simulink model "ultra"  (R2020b)
settings: Solver=FixedStepDiscrete  StartTime=0.0  StopTime=10.0  FixedStep=0.0005  RelTol=1e-3  EnableMultiTasking=on
undefined symbols (not defined in the file): acc_calmax1, acc_calmax2, acc_calmin1, acc_calmin2, akemancanshu, bre, bre_calmax, bre_calmin, ecucoder_acal, I_AN01_5K1, I_AN03_5V, I_AN04_5V, kd, ki, kp, leftmax, O_SW06_HS1A, rightmax, T_add, T_del, tiaoshi, zhiling
libraries: ec5744lib x215, canmsglib x75, simulink x10
(part 3 of 7)

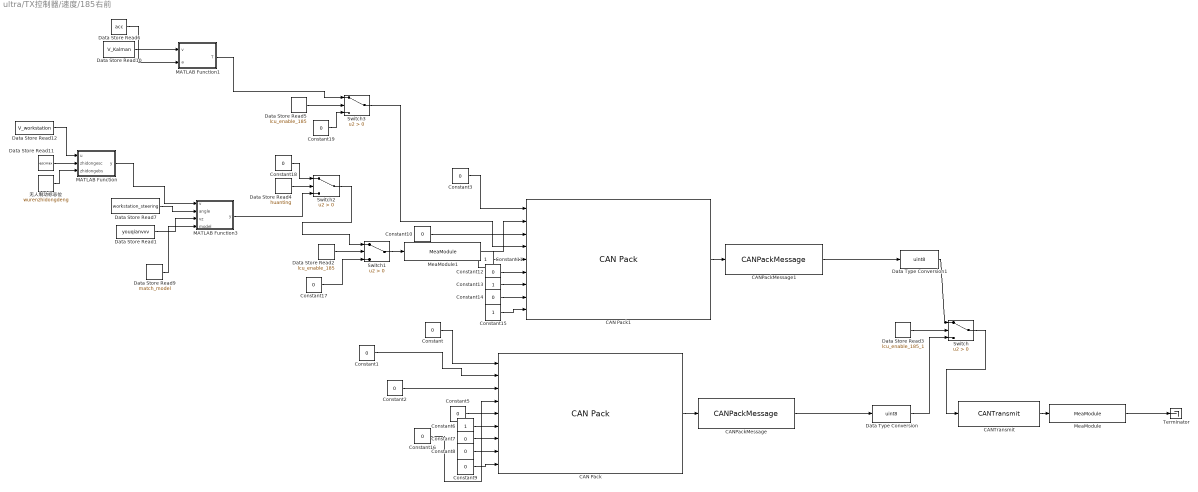
== system ultra/TX控制器/速度/185右前 ==
  CAN Pack : canmsglib/CAN Pack  CANdbFile=D:\desktop\CANdbc\enable - youqian.dbc  MsgList=(none)  MsgName=first_enable  MsgIDType=Standard (11-bit identifier)  MsgIdentifier=389  MsgLength=8  Remote=off  ApplyMinMax=off  BusOutput=off  SignalInfo={'AMK_Reserve','12','4','LE','signed','Standard','0','1','0','0','15';'AMK_TargetVelocity','16','16','LE','signed','Standard','0','1','0','0','65535';'AMK_TorqueLimitNegativ','48','16','LE','signed','Standard','0','1','0','0','65535';'AMK_TorqueLimitPositiv','32','16','LE','signed','Standard','0','1','0','0','65535';'AMK_bEnable','10','1','LE','unsigned','Standard','0','1','0','0','1';'AMK_bErrorReset','11','1','LE','unsigned','Standard','0','1','0','0','1';'AMK_bInverterOn','8','1','LE','unsigned','Standard','0','1','0','0','1';'AMK_bReserve','0','8','LE','unsigned','Standard','0','1','0','0','255';'CAN_bdcon','9','1','LE','unsigned','Standard','0','1','0','0','1'}
      settings: SourceProductBaseCode=ME,XP,VN  DataFormat=CANdb specified signals
  CAN Pack1 : canmsglib/CAN Pack  CANdbFile=D:\desktop\CANdbc\enable - youqian.dbc  MsgList=(none)  MsgName=first_enable  MsgIDType=Standard (11-bit identifier)  MsgIdentifier=389  MsgLength=8  Remote=off  ApplyMinMax=off  BusOutput=off  SignalInfo={'AMK_Reserve','12','4','LE','signed','Standard','0','1','0','0','15';'AMK_TargetVelocity','16','16','LE','signed','Standard','0','1','0','0','65535';'AMK_TorqueLimitNegativ','48','16','LE','signed','Standard','0','1','0','0','65535';'AMK_TorqueLimitPositiv','32','16','LE','signed','Standard','0','1','0','0','65535';'AMK_bEnable','10','1','LE','unsigned','Standard','0','1','0','0','1';'AMK_bErrorReset','11','1','LE','unsigned','Standard','0','1','0','0','1';'AMK_bInverterOn','8','1','LE','unsigned','Standard','0','1','0','0','1';'AMK_bReserve','0','8','LE','unsigned','Standard','0','1','0','0','255';'CAN_bdcon','9','1','LE','unsigned','Standard','0','1','0','0','1'}
      settings: SourceProductBaseCode=ME,XP,VN  DataFormat=CANdb specified signals
  CANPackMessage : ec5744lib/RapidECU_U4B/04CANCommunication/CANPackMessage  datalength=8  sampletime=-1
      settings: SourceProductName=ECUCoder for MPC5744
  CANPackMessage1 : ec5744lib/RapidECU_U4B/04CANCommunication/CANPackMessage  datalength=8  sampletime=-1
      settings: SourceProductName=ECUCoder for MPC5744
  CANTransmit : ec5744lib/RapidECU_U4B/04CANCommunication/CANTransmit  canmodule=0  canbuffer=11  canmessageid=hex2dec('185')  canmessagetype=Standard(11-bit ID)  datalength=8  sampletime=-1
      settings: SourceProductName=ECUCoder for MPC5744
  Constant{,1..3,5,7..10,12,14,16..17,19} (14 alike) : Constant  Value=0  SampleTime=-1
  Constant{6,11,13,15} (4 alike) : Constant  SampleTime=-1
  Constant18 : Constant  Value=0
  Data Store Read1 : DataStoreRead  DataStoreName=youqianvvv
  Data Store Read10 : DataStoreRead  DataStoreName=V_Kalman
  Data Store Read11 : DataStoreRead  DataStoreName=escmax
  Data Store Read12 : DataStoreRead  DataStoreName=V_workstation
  Data Store Read2 : DataStoreRead  DataStoreName=lcu_enable_185
  Data Store Read3 : DataStoreRead  DataStoreName=lcu_enable_185_1
  Data Store Read4 : DataStoreRead  DataStoreName=huanting
  Data Store Read5 : DataStoreRead  DataStoreName=lcu_enable_185
  Data Store Read6 : DataStoreRead  DataStoreName=acc
  Data Store Read7 : DataStoreRead  DataStoreName=workstation_steering
  Data Store Read9 : DataStoreRead  DataStoreName=match_model
  Data Type Conversion : DataTypeConversion  OutDataTypeStr=uint8
  Data Type Conversion1 : DataTypeConversion  OutDataTypeStr=uint8
  MATLAB Function : MATLAB Function  TreatAsAtomicUnit=on
  MATLAB Function1 : MATLAB Function  TreatAsAtomicUnit=on
  MATLAB Function3 : MATLAB Function  TreatAsAtomicUnit=on
  MeaModule : ec5744lib/RapidECU_U4B/07Calibration/MeaModule  signal=V185
      settings: SourceProductName=ECUCoder for MPC5744
  MeaModule1 : ec5744lib/RapidECU_U4B/07Calibration/MeaModule  signal=Vforth
      settings: SourceProductName=ECUCoder for MPC5744
  Switch{,1..3} (4 alike) : Switch  Criteria=u2 > Threshold
  Terminator : Terminator
  无人制动标志位 : DataStoreRead  DataStoreName=wurenzhidongdeng
  wires:
  Constant8/1 -> CAN Pack/8
  Constant5/1 -> CAN Pack/5
  Constant/1 -> CAN Pack/1
  CANPackMessage/1 -> Data Type Conversion/1
  Constant9/1 -> CAN Pack/9
  CAN Pack/1 -> CANPackMessage/1
  Constant7/1 -> CAN Pack/7
  Constant1/1 -> CAN Pack/2
  Constant16/1 -> CAN Pack/4
  Constant2/1 -> CAN Pack/3
  Constant6/1 -> CAN Pack/6
  CANTransmit/1 -> MeaModule/1
  MeaModule/1 -> Terminator/1
  CANPackMessage1/1 -> Data Type Conversion1/1
  Constant3/1 -> CAN Pack1/1
  Constant11/1 -> CAN Pack1/5
  Constant12/1 -> CAN Pack1/6
  Constant13/1 -> CAN Pack1/7
  CAN Pack1/1 -> CANPackMessage1/1
  Constant10/1 -> CAN Pack1/3
  Constant14/1 -> CAN Pack1/8
  Constant15/1 -> CAN Pack1/9
  Data Type Conversion1/1 -> Switch/1
  Data Type Conversion/1 -> Switch/3
  Switch/1 -> CANTransmit/1
  Data Store Read3/1 -> Switch/2
  Switch1/1 -> MeaModule1/1
  Constant17/1 -> Switch1/3
  Data Store Read2/1 -> Switch1/2
  Data Store Read4/1 -> Switch2/2
  Constant18/1 -> Switch2/1
  Switch2/1 -> Switch1/1
  MeaModule1/1 -> CAN Pack1/2
  Constant19/1 -> Switch3/3
  Switch3/1 -> CAN Pack1/4
  Data Store Read5/1 -> Switch3/2
  Data Store Read7/1 -> MATLAB Function3/2(angle)
  Data Store Read1/1 -> MATLAB Function3/3(vz)
  MATLAB Function3/1(y) -> Switch2/3
  Data Store Read9/1 -> MATLAB Function3/4(model)
  MATLAB Function1/1(T) -> Switch3/1
  Data Store Read6/1 -> MATLAB Function1/2(a)
  Data Store Read10/1 -> MATLAB Function1/1(v)
  无人制动标志位/1 -> MATLAB Function/3(zhidongebs)
  MATLAB Function/1(y) -> MATLAB Function3/1(v)
  Data Store Read11/1 -> MATLAB Function/2(zhidongesc)
  Data Store Read12/1 -> MATLAB Function/1(u)

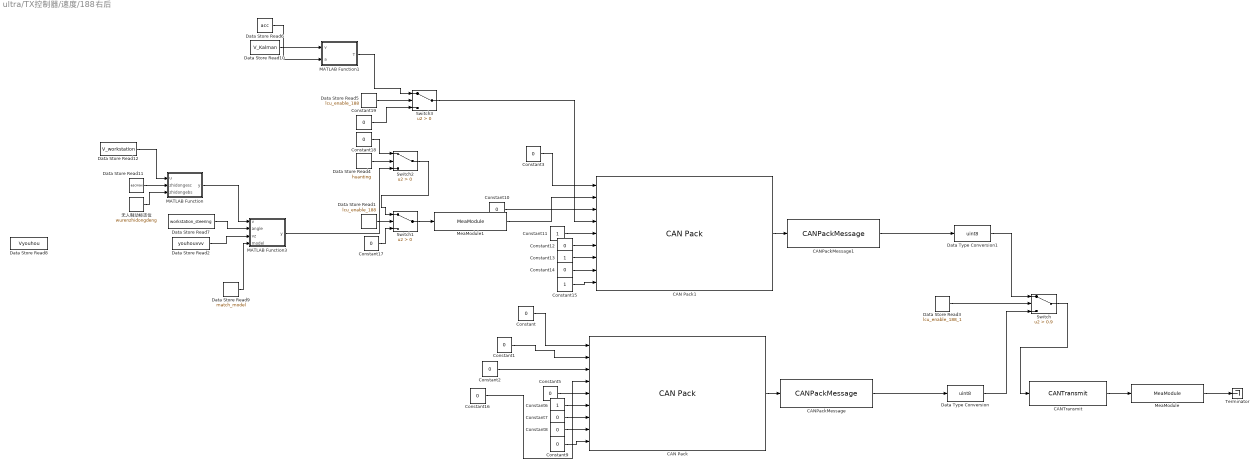
== system ultra/TX控制器/速度/188右后 ==
  CAN Pack : canmsglib/CAN Pack  CANdbFile=D:\desktop\CANdbc\enable - zuohou - 副本.dbc  MsgList=(none)  MsgName=first_enable  MsgIDType=Standard (11-bit identifier)  MsgIdentifier=392  MsgLength=8  Remote=off  ApplyMinMax=off  BusOutput=off  SignalInfo={'AMK_Reserve','12','4','LE','signed','Standard','0','1','0','0','15';'AMK_TargetVelocity','16','16','LE','signed','Standard','0','1','0','0','65535';'AMK_TorqueLimitNegativ','48','16','LE','signed','Standard','0','1','0','0','65535';'AMK_TorqueLimitPositiv','32','16','LE','signed','Standard','0','1','0','0','65535';'AMK_bEnable','10','1','LE','unsigned','Standard','0','1','0','0','1';'AMK_bErrorReset','11','1','LE','unsigned','Standard','0','1','0','0','1';'AMK_bInverterOn','8','1','LE','unsigned','Standard','0','1','0','0','1';'AMK_bReserve','0','8','LE','unsigned','Standard','0','1','0','0','255';'CAN_bdcon','9','1','LE','unsigned','Standard','0','1','0','0','1'}
      settings: SourceProductBaseCode=ME,XP,VN  DataFormat=CANdb specified signals
  CAN Pack1 : canmsglib/CAN Pack  CANdbFile=D:\desktop\CANdbc\enable - zuohou - 副本.dbc  MsgList=(none)  MsgName=first_enable  MsgIDType=Standard (11-bit identifier)  MsgIdentifier=392  MsgLength=8  Remote=off  ApplyMinMax=off  BusOutput=off  SignalInfo={'AMK_Reserve','12','4','LE','signed','Standard','0','1','0','0','15';'AMK_TargetVelocity','16','16','LE','signed','Standard','0','1','0','0','65535';'AMK_TorqueLimitNegativ','48','16','LE','signed','Standard','0','1','0','0','65535';'AMK_TorqueLimitPositiv','32','16','LE','signed','Standard','0','1','0','0','65535';'AMK_bEnable','10','1','LE','unsigned','Standard','0','1','0','0','1';'AMK_bErrorReset','11','1','LE','unsigned','Standard','0','1','0','0','1';'AMK_bInverterOn','8','1','LE','unsigned','Standard','0','1','0','0','1';'AMK_bReserve','0','8','LE','unsigned','Standard','0','1','0','0','255';'CAN_bdcon','9','1','LE','unsigned','Standard','0','1','0','0','1'}
      settings: SourceProductBaseCode=ME,XP,VN  DataFormat=CANdb specified signals
  CANPackMessage : ec5744lib/RapidECU_U4B/04CANCommunication/CANPackMessage  datalength=8  sampletime=-1
      settings: SourceProductName=ECUCoder for MPC5744
  CANPackMessage1 : ec5744lib/RapidECU_U4B/04CANCommunication/CANPackMessage  datalength=8  sampletime=-1
      settings: SourceProductName=ECUCoder for MPC5744
  CANTransmit : ec5744lib/RapidECU_U4B/04CANCommunication/CANTransmit  canmodule=0  canbuffer=9  canmessageid=hex2dec('188')  canmessagetype=Standard(11-bit ID)  datalength=8  sampletime=-1
      settings: SourceProductName=ECUCoder for MPC5744
  Constant{,1..3,5,7..10,12,14,17,19} (13 alike) : Constant  Value=0  SampleTime=-1
  Constant{6,11,13,15} (4 alike) : Constant  SampleTime=-1
  Constant16 : Constant  Value=0
  Constant18 : Constant  Value=0
  Data Store Read1 : DataStoreRead  DataStoreName=lcu_enable_188
  Data Store Read10 : DataStoreRead  DataStoreName=V_Kalman
  Data Store Read11 : DataStoreRead  DataStoreName=escmax
  Data Store Read12 : DataStoreRead  DataStoreName=V_workstation
  Data Store Read2 : DataStoreRead  DataStoreName=youhouvvv
  Data Store Read3 : DataStoreRead  DataStoreName=lcu_enable_188_1
  Data Store Read4 : DataStoreRead  DataStoreName=huanting
  Data Store Read5 : DataStoreRead  DataStoreName=lcu_enable_188
  Data Store Read6 : DataStoreRead  DataStoreName=acc
  Data Store Read7 : DataStoreRead  DataStoreName=workstation_steering
  Data Store Read8 : DataStoreRead  DataStoreName=Vyouhou
  Data Store Read9 : DataStoreRead  DataStoreName=match_model
  Data Type Conversion : DataTypeConversion  OutDataTypeStr=uint8
  Data Type Conversion1 : DataTypeConversion  OutDataTypeStr=uint8
  MATLAB Function : MATLAB Function  TreatAsAtomicUnit=on
  MATLAB Function1 : MATLAB Function  TreatAsAtomicUnit=on
  MATLAB Function3 : MATLAB Function  TreatAsAtomicUnit=on
  MeaModule : ec5744lib/RapidECU_U4B/07Calibration/MeaModule  signal=V188
      settings: SourceProductName=ECUCoder for MPC5744
  MeaModule1 : ec5744lib/RapidECU_U4B/07Calibration/MeaModule  signal=Vsecond
      settings: SourceProductName=ECUCoder for MPC5744
  Switch : Switch  Criteria=u2 > Threshold  Threshold=0.9
  Switch1 : Switch  Criteria=u2 > Threshold
  Switch2 : Switch  Criteria=u2 > Threshold
  Switch3 : Switch  Criteria=u2 > Threshold
  Terminator : Terminator
  无人制动标志位 : DataStoreRead  DataStoreName=wurenzhidongdeng
  wires:
  Constant8/1 -> CAN Pack/8
  Constant5/1 -> CAN Pack/5
  Constant/1 -> CAN Pack/1
  CANPackMessage/1 -> Data Type Conversion/1
  Constant9/1 -> CAN Pack/9
  CAN Pack/1 -> CANPackMessage/1
  Constant7/1 -> CAN Pack/7
  Constant1/1 -> CAN Pack/2
  Constant16/1 -> CAN Pack/4
  Constant2/1 -> CAN Pack/3
  Constant6/1 -> CAN Pack/6
  CANTransmit/1 -> MeaModule/1
  MeaModule/1 -> Terminator/1
  Data Type Conversion1/1 -> Switch/1
  Constant12/1 -> CAN Pack1/6
  Constant10/1 -> CAN Pack1/3
  CANPackMessage1/1 -> Data Type Conversion1/1
  Constant14/1 -> CAN Pack1/8
  Constant3/1 -> CAN Pack1/1
  Constant11/1 -> CAN Pack1/5
  CAN Pack1/1 -> CANPackMessage1/1
  Constant15/1 -> CAN Pack1/9
  Constant13/1 -> CAN Pack1/7
  Data Store Read3/1 -> Switch/2
  Data Type Conversion/1 -> Switch/3
  Switch/1 -> CANTransmit/1
  Constant17/1 -> Switch1/3
  Data Store Read1/1 -> Switch1/2
  Switch1/1 -> MeaModule1/1
  Data Store Read4/1 -> Switch2/2
  Constant18/1 -> Switch2/1
  Switch2/1 -> Switch1/1
  MeaModule1/1 -> CAN Pack1/2
  Switch3/1 -> CAN Pack1/4
  Constant19/1 -> Switch3/3
  Data Store Read5/1 -> Switch3/2
  Data Store Read7/1 -> MATLAB Function3/2(angle)
  MATLAB Function3/1(y) -> Switch2/3
  Data Store Read9/1 -> MATLAB Function3/4(model)
  Data Store Read10/1 -> MATLAB Function1/1(v)
  Data Store Read6/1 -> MATLAB Function1/2(a)
  MATLAB Function1/1(T) -> Switch3/1
  无人制动标志位/1 -> MATLAB Function/3(zhidongebs)
  MATLAB Function/1(y) -> MATLAB Function3/1(v)
  Data Store Read11/1 -> MATLAB Function/2(zhidongesc)
  Data Store Read12/1 -> MATLAB Function/1(u)
  Data Store Read2/1 -> MATLAB Function3/3(vz)

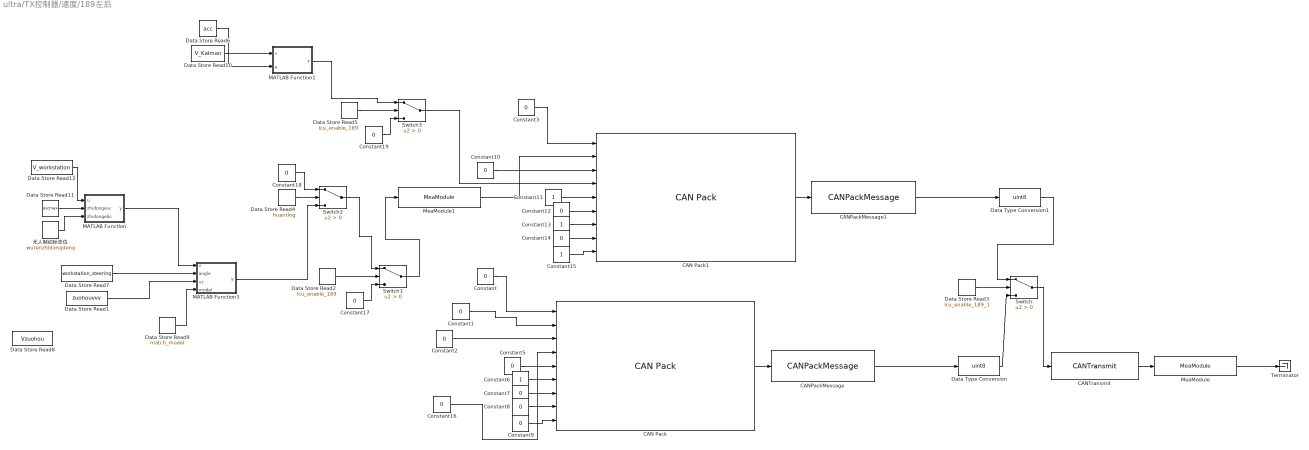
== system ultra/TX控制器/速度/189左后 ==
  CAN Pack : canmsglib/CAN Pack  CANdbFile=D:\desktop\CANdbc\enable - youhou -.dbc  MsgList=(none)  MsgName=first_enable  MsgIDType=Standard (11-bit identifier)  MsgIdentifier=393  MsgLength=8  Remote=off  ApplyMinMax=off  BusOutput=off  SignalInfo={'AMK_Reserve','12','4','LE','signed','Standard','0','1','0','0','15';'AMK_TargetVelocity','16','16','LE','signed','Standard','0','1','0','0','65535';'AMK_TorqueLimitNegativ','48','16','LE','signed','Standard','0','1','0','0','65535';'AMK_TorqueLimitPositiv','32','16','LE','signed','Standard','0','1','0','0','65535';'AMK_bEnable','10','1','LE','unsigned','Standard','0','1','0','0','1';'AMK_bErrorReset','11','1','LE','unsigned','Standard','0','1','0','0','1';'AMK_bInverterOn','8','1','LE','unsigned','Standard','0','1','0','0','1';'AMK_bReserve','0','8','LE','unsigned','Standard','0','1','0','0','255';'CAN_bdcon','9','1','LE','unsigned','Standard','0','1','0','0','1'}
      settings: SourceProductBaseCode=ME,XP,VN  DataFormat=CANdb specified signals
  CAN Pack1 : canmsglib/CAN Pack  CANdbFile=D:\desktop\CANdbc\enable - youhou -.dbc  MsgList=(none)  MsgName=first_enable  MsgIDType=Standard (11-bit identifier)  MsgIdentifier=393  MsgLength=8  Remote=off  ApplyMinMax=off  BusOutput=off  SignalInfo={'AMK_Reserve','12','4','LE','signed','Standard','0','1','0','0','15';'AMK_TargetVelocity','16','16','LE','signed','Standard','0','1','0','0','65535';'AMK_TorqueLimitNegativ','48','16','LE','signed','Standard','0','1','0','0','65535';'AMK_TorqueLimitPositiv','32','16','LE','signed','Standard','0','1','0','0','65535';'AMK_bEnable','10','1','LE','unsigned','Standard','0','1','0','0','1';'AMK_bErrorReset','11','1','LE','unsigned','Standard','0','1','0','0','1';'AMK_bInverterOn','8','1','LE','unsigned','Standard','0','1','0','0','1';'AMK_bReserve','0','8','LE','unsigned','Standard','0','1','0','0','255';'CAN_bdcon','9','1','LE','unsigned','Standard','0','1','0','0','1'}
      settings: SourceProductBaseCode=ME,XP,VN  DataFormat=CANdb specified signals
  CANPackMessage : ec5744lib/RapidECU_U4B/04CANCommunication/CANPackMessage  datalength=8  sampletime=-1
      settings: SourceProductName=ECUCoder for MPC5744
  CANPackMessage1 : ec5744lib/RapidECU_U4B/04CANCommunication/CANPackMessage  datalength=8  sampletime=-1
      settings: SourceProductName=ECUCoder for MPC5744
  CANTransmit : ec5744lib/RapidECU_U4B/04CANCommunication/CANTransmit  canmodule=0  canbuffer=10  canmessageid=hex2dec('189')  canmessagetype=Standard(11-bit ID)  datalength=8  sampletime=-1
      settings: SourceProductName=ECUCoder for MPC5744
  Constant{,1..3,5,7..10,12,14,16..17,19} (14 alike) : Constant  Value=0  SampleTime=-1
  Constant{6,11,13,15} (4 alike) : Constant  SampleTime=-1
  Constant18 : Constant  Value=0
  Data Store Read1 : DataStoreRead  DataStoreName=zuohouvvv
  Data Store Read10 : DataStoreRead  DataStoreName=V_Kalman
  Data Store Read11 : DataStoreRead  DataStoreName=escmax
  Data Store Read12 : DataStoreRead  DataStoreName=V_workstation
  Data Store Read2 : DataStoreRead  DataStoreName=lcu_enable_189
  Data Store Read3 : DataStoreRead  DataStoreName=lcu_enable_189_1
  Data Store Read4 : DataStoreRead  DataStoreName=huanting
  Data Store Read5 : DataStoreRead  DataStoreName=lcu_enable_189
  Data Store Read6 : DataStoreRead  DataStoreName=acc
  Data Store Read7 : DataStoreRead  DataStoreName=workstation_steering
  Data Store Read8 : DataStoreRead  DataStoreName=Vzuohou
  Data Store Read9 : DataStoreRead  DataStoreName=match_model
  Data Type Conversion : DataTypeConversion  OutDataTypeStr=uint8
  Data Type Conversion1 : DataTypeConversion  OutDataTypeStr=uint8
  MATLAB Function : MATLAB Function  TreatAsAtomicUnit=on
  MATLAB Function1 : MATLAB Function  TreatAsAtomicUnit=on
  MATLAB Function3 : MATLAB Function  TreatAsAtomicUnit=on
  MeaModule : ec5744lib/RapidECU_U4B/07Calibration/MeaModule  signal=V189
      settings: SourceProductName=ECUCoder for MPC5744
  MeaModule1 : ec5744lib/RapidECU_U4B/07Calibration/MeaModule  signal=Vthird
      settings: SourceProductName=ECUCoder for MPC5744
  Switch{,1..3} (4 alike) : Switch  Criteria=u2 > Threshold
  Terminator : Terminator
  无人制动标志位 : DataStoreRead  DataStoreName=wurenzhidongdeng
  wires:
  Constant8/1 -> CAN Pack/8
  Constant5/1 -> CAN Pack/5
  Constant/1 -> CAN Pack/1
  CANPackMessage/1 -> Data Type Conversion/1
  Constant9/1 -> CAN Pack/9
  CAN Pack/1 -> CANPackMessage/1
  Constant7/1 -> CAN Pack/7
  Constant1/1 -> CAN Pack/2
  Constant16/1 -> CAN Pack/4
  Constant2/1 -> CAN Pack/3
  Constant6/1 -> CAN Pack/6
  CANTransmit/1 -> MeaModule/1
  MeaModule/1 -> Terminator/1
  Constant12/1 -> CAN Pack1/6
  Constant10/1 -> CAN Pack1/3
  Constant14/1 -> CAN Pack1/8
  Constant11/1 -> CAN Pack1/5
  Constant13/1 -> CAN Pack1/7
  CANPackMessage1/1 -> Data Type Conversion1/1
  CAN Pack1/1 -> CANPackMessage1/1
  Constant15/1 -> CAN Pack1/9
  Constant3/1 -> CAN Pack1/1
  Data Type Conversion1/1 -> Switch/1
  Data Type Conversion/1 -> Switch/3
  Switch/1 -> CANTransmit/1
  Data Store Read3/1 -> Switch/2
  Constant17/1 -> Switch1/3
  Data Store Read2/1 -> Switch1/2
  Switch1/1 -> MeaModule1/1
  Data Store Read4/1 -> Switch2/2
  Constant18/1 -> Switch2/1
  Switch2/1 -> Switch1/1
  MeaModule1/1 -> CAN Pack1/2
  Constant19/1 -> Switch3/3
  Switch3/1 -> CAN Pack1/4
  Data Store Read5/1 -> Switch3/2
  Data Store Read7/1 -> MATLAB Function3/2(angle)
  MATLAB Function3/1(y) -> Switch2/3
  MATLAB Function/1(y) -> MATLAB Function3/1(v)
  Data Store Read9/1 -> MATLAB Function3/4(model)
  Data Store Read6/1 -> MATLAB Function1/2(a)
  Data Store Read10/1 -> MATLAB Function1/1(v)
  MATLAB Function1/1(T) -> Switch3/1
  无人制动标志位/1 -> MATLAB Function/3(zhidongebs)
  Data Store Read11/1 -> MATLAB Function/2(zhidongesc)
  Data Store Read12/1 -> MATLAB Function/1(u)
  Data Store Read1/1 -> MATLAB Function3/3(vz)

== system ultra/run/analog_input/无人意图转译 ==
  note: 输出基准转矩
  Enable : EnablePort
  Data Store Read : DataStoreRead  DataStoreName=CANOK_20
  Saturation : Saturate  UpperLimit=1300  LowerLimit=0
  无人 : Subsystem
  计算期望扭矩 : MATLAB Function  TreatAsAtomicUnit=on
  Out1 : Outport
  wires:
  无人/1(期望纵向加速度) -> 计算期望扭矩/1(u)
  计算期望扭矩/1(y) -> Saturation/1
  Saturation/1 -> Out1/1
  Data Store Read/1 -> 计算期望扭矩/2(canok)

== system ultra/run/analog_input/有人 ==
  note: 加速踏板信号转化为0-1范围
      | 即开度
  Enable : EnablePort
  Data Store Write : DataStoreWrite  DataStoreName=yourenniuju
  MeaModule9 : ec5744lib/RapidECU_U4B/07Calibration/MeaModule  signal=tttttttt
      settings: SourceProductName=ECUCoder for MPC5744
  Subsystem : Subsystem
  Subsystem1 : Subsystem
  TP : Outport
  bre : Outport  Port=2
  wires:
  Subsystem/2(bre) -> bre/1
  Subsystem/1(acc) -> Subsystem1/1(acc_signal)
  Subsystem1/1(TP) -> MeaModule9/1
  MeaModule9/1 -> Data Store Write/1, TP/1

== system ultra/run/ctrl/Subsystem1 ==
  扭矩 : Inport
  Data Store Write : DataStoreWrite  DataStoreName=Tzuoqian
  Data Store Write1 : DataStoreWrite  DataStoreName=Tyouhou
  Data Store Write2 : DataStoreWrite  DataStoreName=Tzuohou
  Data Store Write3 : DataStoreWrite  DataStoreName=Tyouqian
  control_strategy : Subsystem
  wires:
  control_strategy/3(zuohou) -> Data Store Write2/1
  扭矩/1 -> control_strategy/1(TP)
  control_strategy/2(youqian) -> Data Store Write3/1
  control_strategy/1(youhou) -> Data Store Write1/1
  control_strategy/4(zuoqian) -> Data Store Write/1

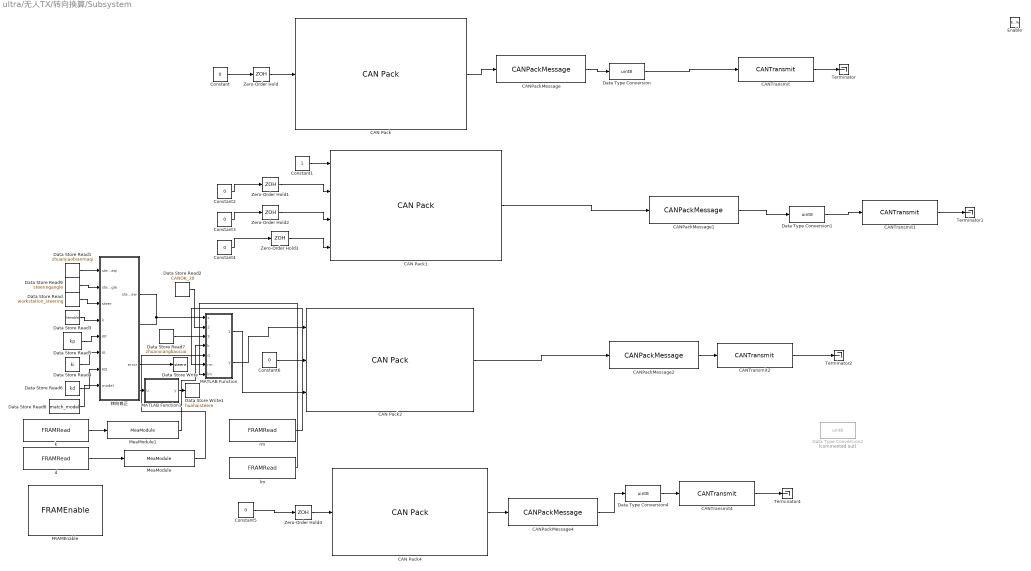
== system ultra/无人TX/转向换算/Subsystem ==
  Enable : EnablePort
  CAN Pack : canmsglib/CAN Pack  CANdbFile=C:\Users\Liu keliang\Desktop\HRT2023\HRT23赛季刘科良\CANdbc\steering.dbc  MsgList=enable123  MsgName=enable123  MsgIDType=Standard (11-bit identifier)  MsgIdentifier=291  MsgLength=1  Remote=off  ApplyMinMax=off  BusOutput=off  SignalInfo={'enable123','0','8','LE','unsigned','Standard','0','1','0','0','255'}
      settings: SourceProductBaseCode=ME,XP,VN  DataFormat=CANdb specified signals
  CAN Pack1 : canmsglib/CAN Pack  CANdbFile=C:\Users\Liu keliang\Desktop\HRT2023\HRT23赛季刘科良\CANdbc\steering.dbc  MsgList=enable0  MsgName=enable0  MsgIDType=Standard (11-bit identifier)  MsgIdentifier=0  MsgLength=8  Remote=off  ApplyMinMax=off  BusOutput=off  SignalInfo={'enable_00','0','16','LE','unsigned','Standard','0','1','0','0','65535';'enable_00_Copy_1','16','16','LE','unsigned','Standard','0','1','0','0','65535';'enable_00_Copy_2','32','16','LE','unsigned','Standard','0','1','0','0','65535';'enable_00_Copy_3','48','16','LE','unsigned','Standard','0','1','0','0','65535'}
      settings: SourceProductBaseCode=ME,XP,VN  DataFormat=CANdb specified signals
  CAN Pack2 : canmsglib/CAN Pack  CANdbFile=C:\Users\Liu keliang\Desktop\HRT2023\HRT23赛季刘科良\CANdbc\steering.dbc  MsgList=enable401  MsgName=enable401  MsgIDType=Standard (11-bit identifier)  MsgIdentifier=1025  MsgLength=6  Remote=off  ApplyMinMax=off  BusOutput=off  SignalInfo={'enable401','0','8','LE','unsigned','Standard','0','1','0','0','255';'enable401_Copy_1','8','8','LE','unsigned','Standard','0','1','0','0','255';'enable401_Copy_2','16','32','LE','signed','Standard','0','1','0','-2147483648','2147483647'}
      settings: SourceProductBaseCode=ME,XP,VN  DataFormat=CANdb specified signals
  CAN Pack4 : canmsglib/CAN Pack  CANdbFile=C:\Users\Liu keliang\Desktop\HRT2023\HRT23赛季刘科良\CANdbc\steering.dbc  MsgList=enable80  MsgName=enable80  MsgIDType=Standard (11-bit identifier)  MsgIdentifier=128  MsgLength=1  Remote=off  ApplyMinMax=off  BusOutput=off  SignalInfo={'dingshi','0','8','LE','unsigned','Standard','0','1','0','0','255'}
      settings: SourceProductBaseCode=ME,XP,VN  DataFormat=CANdb specified signals
  CANPackMessage : ec5744lib/RapidECU_U4B/04CANCommunication/CANPackMessage  datalength=1  sampletime=-1
      settings: SourceProductName=ECUCoder for MPC5744
  CANPackMessage1 : ec5744lib/RapidECU_U4B/04CANCommunication/CANPackMessage  datalength=8  sampletime=-1
      settings: SourceProductName=ECUCoder for MPC5744
  CANPackMessage2 : ec5744lib/RapidECU_U4B/04CANCommunication/CANPackMessage  datalength=6  sampletime=-1
      settings: SourceProductName=ECUCoder for MPC5744
  CANPackMessage4 : ec5744lib/RapidECU_U4B/04CANCommunication/CANPackMessage  datalength=1  sampletime=-1
      settings: SourceProductName=ECUCoder for MPC5744
  CANTransmit : ec5744lib/RapidECU_U4B/04CANCommunication/CANTransmit  canmodule=1  canbuffer=15  canmessageid=hex2dec('123')  canmessagetype=Standard(11-bit ID)  datalength=1  sampletime=-1
      settings: SourceProductName=ECUCoder for MPC5744
  CANTransmit1 : ec5744lib/RapidECU_U4B/04CANCommunication/CANTransmit  canmodule=1  canbuffer=56  canmessageid=hex2dec('00')  canmessagetype=Standard(11-bit ID)  datalength=8  sampletime=-1
      settings: SourceProductName=ECUCoder for MPC5744
  CANTransmit2 : ec5744lib/RapidECU_U4B/04CANCommunication/CANTransmit  canmodule=1  canbuffer=57  canmessageid=hex2dec('401')  canmessagetype=Standard(11-bit ID)  datalength=6  sampletime=-1
      settings: SourceProductName=ECUCoder for MPC5744
  CANTransmit4 : ec5744lib/RapidECU_U4B/04CANCommunication/CANTransmit  canmodule=1  canbuffer=58  canmessageid=hex2dec('80')  canmessagetype=Standard(11-bit ID)  datalength=1  sampletime=-1
      settings: SourceProductName=ECUCoder for MPC5744
  Constant : Constant  Value=0  SampleTime=-1
  Constant1 : Constant  SampleTime=-1
  Constant{2..4,6} (4 alike) : Constant  Value=0
  Constant5 : Constant  Value=0  SampleTime=-1
  Data Store Read : DataStoreRead  DataStoreName=workstation_steering
  Data Store Read1 : DataStoreRead  DataStoreName=zhuanjiaobianmaqi
  Data Store Read2 : DataStoreRead  DataStoreName=CANOK_20
  Data Store Read3 : DataStoreRead  DataStoreName=kenable
  Data Store Read4 : DataStoreRead  DataStoreName=ki
  Data Store Read5 : DataStoreRead  DataStoreName=kp
  Data Store Read6 : DataStoreRead  DataStoreName=kd
  Data Store Read7 : DataStoreRead  DataStoreName=zhuanxiangbaocuo
  Data Store Read8 : DataStoreRead  DataStoreName=match_model
  Data Store Read9 : DataStoreRead  DataStoreName=steeringangle
  Data Store Write : DataStoreWrite  DataStoreName=steere
  Data Store Write1 : DataStoreWrite  DataStoreName=huahaisteere
  Data Type Conversion : DataTypeConversion  OutDataTypeStr=uint8
  Data Type Conversion1 : DataTypeConversion  OutDataTypeStr=uint8
  Data Type Conversion2 : DataTypeConversion  Commented=on  OutDataTypeStr=uint8
  Data Type Conversion4 : DataTypeConversion  OutDataTypeStr=uint8
  FRAMEnable : ec5744lib/RapidECU_U4B/12EEModule/FRAMEnable  framenable=on
      settings: SourceProductName=ECUCoder for MPC5744
  MATLAB Function : MATLAB Function  TreatAsAtomicUnit=on
  MATLAB Function1 : MATLAB Function  TreatAsAtomicUnit=on
  MeaModule : ec5744lib/RapidECU_U4B/07Calibration/MeaModule  signal=d
      settings: SourceProductName=ECUCoder for MPC5744
  MeaModule1 : ec5744lib/RapidECU_U4B/07Calibration/MeaModule  signal=k
      settings: SourceProductName=ECUCoder for MPC5744
  Terminator{,1..2,4} (4 alike) : Terminator
  Zero-Order Hold{,1..4} (5 alike) : ZeroOrderHold  SampleTime=-1
  d : ec5744lib/RapidECU_U4B/12EEModule/FRAMRead  buffer=1  sampletime=-1
      settings: SourceProductName=ECUCoder for MPC5744
  k : ec5744lib/RapidECU_U4B/12EEModule/FRAMRead  buffer=0  sampletime=-1
      settings: SourceProductName=ECUCoder for MPC5744
  lm : ec5744lib/RapidECU_U4B/12EEModule/FRAMRead  buffer=11  sampletime=-1
      settings: SourceProductName=ECUCoder for MPC5744
  rm : ec5744lib/RapidECU_U4B/12EEModule/FRAMRead  buffer=10  sampletime=-1
      settings: SourceProductName=ECUCoder for MPC5744
  转向修正 : MATLAB Function  TreatAsAtomicUnit=on
  wires:
  CANTransmit/1 -> Terminator/1
  Zero-Order Hold2/1 -> CAN Pack1/3
  MATLAB Function/2(y) -> CAN Pack2/1
  CAN Pack1/1 -> CANPackMessage1/1
  CANTransmit2/1 -> Terminator2/1
  CANPackMessage4/1 -> Data Type Conversion4/1
  CAN Pack2/1 -> CANPackMessage2/1
  CANTransmit1/1 -> Terminator1/1
  Constant/1 -> Zero-Order Hold/1
  Data Type Conversion1/1 -> CANTransmit1/1
  Constant6/1 -> CAN Pack2/2
  CANTransmit4/1 -> Terminator4/1
  Data Type Conversion/1 -> CANTransmit/1
  Zero-Order Hold/1 -> CAN Pack/1
  CANPackMessage/1 -> Data Type Conversion/1
  Data Type Conversion4/1 -> CANTransmit4/1
  Constant4/1 -> Zero-Order Hold3/1
  CAN Pack/1 -> CANPackMessage/1
  CANPackMessage1/1 -> Data Type Conversion1/1
  Constant5/1 -> Zero-Order Hold4/1
  CAN Pack4/1 -> CANPackMessage4/1
  Constant3/1 -> Zero-Order Hold2/1
  Constant2/1 -> Zero-Order Hold1/1
  Constant1/1 -> CAN Pack1/1
  Zero-Order Hold4/1 -> CAN Pack4/1
  Zero-Order Hold1/1 -> CAN Pack1/2
  CANPackMessage2/1 -> CANTransmit2/1
  Zero-Order Hold3/1 -> CAN Pack1/4
  MATLAB Function/1(steer) -> CAN Pack2/3
  Data Store Read/1 -> 转向修正/3(steer)
  Data Store Read1/1 -> 转向修正/1(steerbianmaqi)
  转向修正/1(steernew) -> MATLAB Function1/1(u), MATLAB Function/1(x)
  转向修正/2(error) -> Data Store Write/1
  Data Store Read2/1 -> MATLAB Function/2(canok)
  Data Store Read5/1 -> 转向修正/5(KP)
  Data Store Read4/1 -> 转向修正/6(KI)
  Data Store Read3/1 -> 转向修正/4(k)
  Data Store Read6/1 -> 转向修正/7(KD)
  MATLAB Function1/1(y) -> Data Store Write1/1
  Data Store Read7/1 -> MATLAB Function/3(baocuo)
  Data Store Read8/1 -> 转向修正/8(model)
  Data Store Read9/1 -> 转向修正/2(steerangle)
  rm/1 -> MATLAB Function/6(rm)
  lm/1 -> MATLAB Function/7(lm)
  d/1 -> MeaModule/1
  MeaModule/1 -> MATLAB Function/5(d)
  k/1 -> MeaModule1/1
  MeaModule1/1 -> MATLAB Function/4(k)

== system ultra/无人TX/转向换算/Subsystem1 ==
  y1 : Inport
  y2 : Inport  Port=2
  Enable : EnablePort
  CAN Pack5 : canmsglib/CAN Pack  CANdbFile=C:\Users\Liu keliang\Desktop\HRT2023\HRT23赛季刘科良\CANdbc\zhuanxiangresetting.dbc  MsgList=reseting  MsgName=reseting  MsgIDType=Standard (11-bit identifier)  MsgIdentifier=1537  MsgLength=8  Remote=off  ApplyMinMax=off  BusOutput=off  SignalInfo={'reseting1','0','32','LE','unsigned','Standard','0','1','0','-Inf','Inf';'reseting2','32','32','LE','unsigned','Standard','0','1','0','-Inf','Inf'}
      settings: SourceProductBaseCode=ME,XP,VN  DataFormat=CANdb specified signals
  CANPackMessage3 : ec5744lib/RapidECU_U4B/04CANCommunication/CANPackMessage  datalength=8  sampletime=-1
      settings: SourceProductName=ECUCoder for MPC5744
  CANTransmit3 : ec5744lib/RapidECU_U4B/04CANCommunication/CANTransmit  canmodule=1  canbuffer=60  canmessageid=hex2dec('601')  canmessagetype=Standard(11-bit ID)  datalength=8  sampletime=-1
      settings: SourceProductName=ECUCoder for MPC5744
  Data Type Conversion3 : DataTypeConversion  OutDataTypeStr=uint8
  Terminator3 : Terminator
  wires:
  CAN Pack5/1 -> CANPackMessage3/1
  y1/1 -> CAN Pack5/1
  CANTransmit3/1 -> Terminator3/1
  Data Type Conversion3/1 -> CANTransmit3/1
  CANPackMessage3/1 -> Data Type Conversion3/1
  y2/1 -> CAN Pack5/2

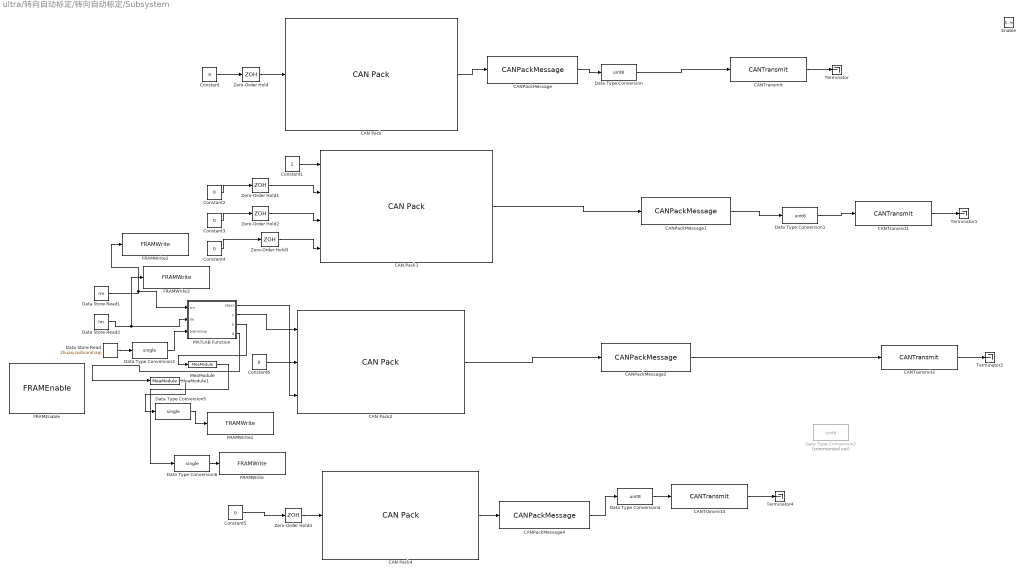
== system ultra/转向自动标定/转向自动标定/Subsystem ==
  Enable : EnablePort
  CAN Pack : canmsglib/CAN Pack  CANdbFile=C:\Users\Liu keliang\Desktop\HRT2023\HRT23赛季刘科良\CANdbc\steering.dbc  MsgList=enable123  MsgName=enable123  MsgIDType=Standard (11-bit identifier)  MsgIdentifier=291  MsgLength=1  Remote=off  ApplyMinMax=off  BusOutput=off  SignalInfo={'enable123','0','8','LE','unsigned','Standard','0','1','0','0','255'}
      settings: SourceProductBaseCode=ME,XP,VN  DataFormat=CANdb specified signals
  CAN Pack1 : canmsglib/CAN Pack  CANdbFile=C:\Users\Liu keliang\Desktop\HRT2023\HRT23赛季刘科良\CANdbc\steering.dbc  MsgList=enable0  MsgName=enable0  MsgIDType=Standard (11-bit identifier)  MsgIdentifier=0  MsgLength=8  Remote=off  ApplyMinMax=off  BusOutput=off  SignalInfo={'enable_00','0','16','LE','unsigned','Standard','0','1','0','0','65535';'enable_00_Copy_1','16','16','LE','unsigned','Standard','0','1','0','0','65535';'enable_00_Copy_2','32','16','LE','unsigned','Standard','0','1','0','0','65535';'enable_00_Copy_3','48','16','LE','unsigned','Standard','0','1','0','0','65535'}
      settings: SourceProductBaseCode=ME,XP,VN  DataFormat=CANdb specified signals
  CAN Pack2 : canmsglib/CAN Pack  CANdbFile=C:\Users\Liu keliang\Desktop\HRT2023\HRT23赛季刘科良\CANdbc\steering.dbc  MsgList=enable401  MsgName=enable401  MsgIDType=Standard (11-bit identifier)  MsgIdentifier=1025  MsgLength=6  Remote=off  ApplyMinMax=off  BusOutput=off  SignalInfo={'enable401','0','8','LE','unsigned','Standard','0','1','0','0','255';'enable401_Copy_1','8','8','LE','unsigned','Standard','0','1','0','0','255';'enable401_Copy_2','16','32','LE','signed','Standard','0','1','0','-2147483648','2147483647'}
      settings: SourceProductBaseCode=ME,XP,VN  DataFormat=CANdb specified signals
  CAN Pack4 : canmsglib/CAN Pack  CANdbFile=C:\Users\Liu keliang\Desktop\HRT2023\HRT23赛季刘科良\CANdbc\steering.dbc  MsgList=enable80  MsgName=enable80  MsgIDType=Standard (11-bit identifier)  MsgIdentifier=128  MsgLength=1  Remote=off  ApplyMinMax=off  BusOutput=off  SignalInfo={'dingshi','0','8','LE','unsigned','Standard','0','1','0','0','255'}
      settings: SourceProductBaseCode=ME,XP,VN  DataFormat=CANdb specified signals
  CANPackMessage : ec5744lib/RapidECU_U4B/04CANCommunication/CANPackMessage  datalength=1  sampletime=-1
      settings: SourceProductName=ECUCoder for MPC5744
  CANPackMessage1 : ec5744lib/RapidECU_U4B/04CANCommunication/CANPackMessage  datalength=8  sampletime=-1
      settings: SourceProductName=ECUCoder for MPC5744
  CANPackMessage2 : ec5744lib/RapidECU_U4B/04CANCommunication/CANPackMessage  datalength=6  sampletime=-1
      settings: SourceProductName=ECUCoder for MPC5744
  CANPackMessage4 : ec5744lib/RapidECU_U4B/04CANCommunication/CANPackMessage  datalength=1  sampletime=-1
      settings: SourceProductName=ECUCoder for MPC5744
  CANTransmit : ec5744lib/RapidECU_U4B/04CANCommunication/CANTransmit  canmodule=1  canbuffer=15  canmessageid=hex2dec('123')  canmessagetype=Standard(11-bit ID)  datalength=1  sampletime=-1
      settings: SourceProductName=ECUCoder for MPC5744
  CANTransmit1 : ec5744lib/RapidECU_U4B/04CANCommunication/CANTransmit  canmodule=1  canbuffer=56  canmessageid=hex2dec('00')  canmessagetype=Standard(11-bit ID)  datalength=8  sampletime=-1
      settings: SourceProductName=ECUCoder for MPC5744
  CANTransmit2 : ec5744lib/RapidECU_U4B/04CANCommunication/CANTransmit  canmodule=1  canbuffer=57  canmessageid=hex2dec('401')  canmessagetype=Standard(11-bit ID)  datalength=6  sampletime=-1
      settings: SourceProductName=ECUCoder for MPC5744
  CANTransmit4 : ec5744lib/RapidECU_U4B/04CANCommunication/CANTransmit  canmodule=1  canbuffer=58  canmessageid=hex2dec('80')  canmessagetype=Standard(11-bit ID)  datalength=1  sampletime=-1
      settings: SourceProductName=ECUCoder for MPC5744
  Constant : Constant  Value=0  SampleTime=-1
  Constant1 : Constant  SampleTime=-1
  Constant{2..4,6} (4 alike) : Constant  Value=0
  Constant5 : Constant  Value=0  SampleTime=-1
  Data Store Read : DataStoreRead  DataStoreName=zhuanjiaobianmaqi
  Data Store Read1 : DataStoreRead  DataStoreName=rm
  Data Store Read2 : DataStoreRead  DataStoreName=lm
  Data Type Conversion : DataTypeConversion  OutDataTypeStr=uint8
  Data Type Conversion1 : DataTypeConversion  OutDataTypeStr=uint8
  Data Type Conversion2 : DataTypeConversion  Commented=on  OutDataTypeStr=uint8
  Data Type Conversion3 : DataTypeConversion  OutDataTypeStr=single
  Data Type Conversion4 : DataTypeConversion  OutDataTypeStr=uint8
  Data Type Conversion5 : DataTypeConversion  OutDataTypeStr=single
  Data Type Conversion6 : DataTypeConversion  OutDataTypeStr=single
  FRAMEnable : ec5744lib/RapidECU_U4B/12EEModule/FRAMEnable  framenable=on
      settings: SourceProductName=ECUCoder for MPC5744
  FRAMWrite : ec5744lib/RapidECU_U4B/12EEModule/FRAMWrite  buffer=0  sampletime=-1
      settings: SourceProductName=ECUCoder for MPC5744
  FRAMWrite1 : ec5744lib/RapidECU_U4B/12EEModule/FRAMWrite  buffer=1  sampletime=-1
      settings: SourceProductName=ECUCoder for MPC5744
  FRAMWrite2 : ec5744lib/RapidECU_U4B/12EEModule/FRAMWrite  buffer=10  sampletime=-1
      settings: SourceProductName=ECUCoder for MPC5744
  FRAMWrite3 : ec5744lib/RapidECU_U4B/12EEModule/FRAMWrite  buffer=11  sampletime=-1
      settings: SourceProductName=ECUCoder for MPC5744
  MATLAB Function : MATLAB Function  TreatAsAtomicUnit=on
  MeaModule : ec5744lib/RapidECU_U4B/07Calibration/MeaModule  signal=msk
      settings: SourceProductName=ECUCoder for MPC5744
  MeaModule1 : ec5744lib/RapidECU_U4B/07Calibration/MeaModule  signal=msd
      settings: SourceProductName=ECUCoder for MPC5744
  Terminator{,1..2,4} (4 alike) : Terminator
  Zero-Order Hold{,1..4} (5 alike) : ZeroOrderHold  SampleTime=-1
  wires:
  CANTransmit/1 -> Terminator/1
  Zero-Order Hold2/1 -> CAN Pack1/3
  MATLAB Function/2(y) -> CAN Pack2/1
  CAN Pack1/1 -> CANPackMessage1/1
  CANTransmit2/1 -> Terminator2/1
  CANPackMessage4/1 -> Data Type Conversion4/1
  CAN Pack2/1 -> CANPackMessage2/1
  CANTransmit1/1 -> Terminator1/1
  Constant/1 -> Zero-Order Hold/1
  Data Type Conversion1/1 -> CANTransmit1/1
  Constant6/1 -> CAN Pack2/2
  CANTransmit4/1 -> Terminator4/1
  Data Type Conversion/1 -> CANTransmit/1
  Zero-Order Hold/1 -> CAN Pack/1
  CANPackMessage/1 -> Data Type Conversion/1
  Data Type Conversion4/1 -> CANTransmit4/1
  Constant4/1 -> Zero-Order Hold3/1
  CAN Pack/1 -> CANPackMessage/1
  CANPackMessage1/1 -> Data Type Conversion1/1
  Constant5/1 -> Zero-Order Hold4/1
  CAN Pack4/1 -> CANPackMessage4/1
  Constant3/1 -> Zero-Order Hold2/1
  Constant2/1 -> Zero-Order Hold1/1
  Constant1/1 -> CAN Pack1/1
  Zero-Order Hold4/1 -> CAN Pack4/1
  Zero-Order Hold1/1 -> CAN Pack1/2
  CANPackMessage2/1 -> CANTransmit2/1
  Zero-Order Hold3/1 -> CAN Pack1/4
  MATLAB Function/1(steer) -> CAN Pack2/3
  Data Store Read/1 -> Data Type Conversion3/1
  MATLAB Function/3(k) -> MeaModule/1
  Data Store Read1/1 -> FRAMWrite2/1, MATLAB Function/1(rm)
  Data Store Read2/1 -> MATLAB Function/2(lm), FRAMWrite3/1
  Data Type Conversion3/1 -> MATLAB Function/3(bianmaqi)
  MATLAB Function/4(d) -> MeaModule1/1
  MeaModule1/1 -> Data Type Conversion5/1
  Data Type Conversion5/1 -> FRAMWrite1/1
  Data Type Conversion6/1 -> FRAMWrite/1
  MeaModule/1 -> Data Type Conversion6/1

== system ultra/转向自动标定/转向自动标定/Subsystem1 ==
  y1 : Inport
  y2 : Inport  Port=2
  Enable : EnablePort
  CAN Pack5 : canmsglib/CAN Pack  CANdbFile=C:\Users\Liu keliang\Desktop\HRT2023\HRT23赛季刘科良\CANdbc\zhuanxiangresetting.dbc  MsgList=reseting  MsgName=reseting  MsgIDType=Standard (11-bit identifier)  MsgIdentifier=1537  MsgLength=8  Remote=off  ApplyMinMax=off  BusOutput=off  SignalInfo={'reseting1','0','32','LE','unsigned','Standard','0','1','0','-Inf','Inf';'reseting2','32','32','LE','unsigned','Standard','0','1','0','-Inf','Inf'}
      settings: SourceProductBaseCode=ME,XP,VN  DataFormat=CANdb specified signals
  CANPackMessage3 : ec5744lib/RapidECU_U4B/04CANCommunication/CANPackMessage  datalength=8  sampletime=-1
      settings: SourceProductName=ECUCoder for MPC5744
  CANTransmit3 : ec5744lib/RapidECU_U4B/04CANCommunication/CANTransmit  canmodule=1  canbuffer=60  canmessageid=hex2dec('601')  canmessagetype=Standard(11-bit ID)  datalength=8  sampletime=-1
      settings: SourceProductName=ECUCoder for MPC5744
  Data Type Conversion3 : DataTypeConversion  OutDataTypeStr=uint8
  Terminator3 : Terminator
  wires:
  CAN Pack5/1 -> CANPackMessage3/1
  y1/1 -> CAN Pack5/1
  CANTransmit3/1 -> Terminator3/1
  Data Type Conversion3/1 -> CANTransmit3/1
  CANPackMessage3/1 -> Data Type Conversion3/1
  y2/1 -> CAN Pack5/2

== system ultra/RX/283 285左前/Subsystem1/Subsystem ==
  ID : Inport
  msg : Inport  Port=2
  Enable : EnablePort
  CAN Pack : canmsglib/CAN Pack  Commented=on  CANdbFile=D:\desktop\enable.dbc  MsgList=(none)  MsgName=AMK_ActualValue1  MsgIDType=Standard (11-bit identifier)  MsgIdentifier=643  MsgLength=8  Remote=off  ApplyMinMax=off  BusOutput=off  SignalInfo={'AMK_ActualVelocity','16','16','LE','signed','Standard','0','1','0','0','65535';'AMK_MagnetizingCurrent','48','16','LE','signed','Standard','0','1','0','0','65535';'AMK_TorqueCurrent','32','16','LE','signed','Standard','0','1','0','0','65535';'AMK_bDcOn1','12','1','LE','unsigned','Standard','0','1','0','0','1';'AMK_bDerating1','15','1','LE','unsigned','Standard','0','1','0','0','1';'AMK_bError1','9','1','LE','unsigned','Standard','0','1','0','0','1';'AMK_bInverterOn1','14','1','LE','unsigned','Standard','0','1','0','0','1';'AMK_bQuitDcOn1','11','1','LE','unsigned','Standard','0','1','0','0','1';'AMK_bQuitInverterOn1','13','1','LE','unsigned','Standard','0','1','0','0','1';'AMK_bReserve1','0','8','LE','unsigned','Standard','0','1','0','0','255';'AMK_bSystemReady1','8','1','LE','unsigned','Standard','0','1','0','0','1';'AMK_bWarn1','10','1','LE','unsigned','Standard','0','1','0','0','1'}
      settings: SourceProductBaseCode=ME,XP,VN  DataFormat=CANdb specified signals
  CAN Unpack : canmsglib/CAN Unpack  CANdbFile=D:\desktop\刘科良\HRT23赛季刘科良\CANdbc\enable.dbc  MsgList=(none)  MsgName=AMK_ActualValue2  MsgIDType=Standard (11-bit identifier)  MsgIdentifier=645  MsgLength=8  SignalInfo={'AMK_ErrorInfo','32','16','LE','unsigned','Standard','0','1','0','0','65535';'AMK_TempIGBT','48','16','LE','signed','Standard','0','1','0','0','65535';'AMK_TempInverter','16','16','LE','signed','Standard','0','1','0','-32768','32767';'AMK_TempMotor','0','16','LE','signed','Standard','0','1','0','0','65535'}  IDPort=off  TimestampPort=off  ErrorPort=off  RemotePort=off  LengthPort=off  StatusPort=off  ApplyMinMax=off
      settings: SourceProductBaseCode=ME,XP,VN  DataFormat=CANdb specified signals
  CANPackMessage : ec5744lib/RapidECU_U4B/04CANCommunication/CANPackMessage  Commented=on  datalength=8  sampletime=-1
      settings: SourceProductName=ECUCoder for MPC5744
  CANUnPackMessage : ec5744lib/RapidECU_U4B/04CANCommunication/CANUnPackMessage  datalength=8  canmessagetype=Standard(11-bit ID)  sampletime=-1
      settings: SourceProductName=ECUCoder for MPC5744
  wires:
  msg/1 -> CANUnPackMessage/2
  CANUnPackMessage/1 -> CAN Unpack/1
  ID/1 -> CANUnPackMessage/1
  CANPackMessage/1 -> ?
  CAN Pack/1 -> CANPackMessage/1

== system ultra/RX/283 285左前/Subsystem2/Subsystem ==
  ID : Inport
  msg : Inport  Port=2
  Enable : EnablePort
  CAN Pack : canmsglib/CAN Pack  Commented=on  CANdbFile=D:\desktop\enable.dbc  MsgList=(none)  MsgName=AMK_ActualValue1  MsgIDType=Standard (11-bit identifier)  MsgIdentifier=643  MsgLength=8  Remote=off  ApplyMinMax=off  BusOutput=off  SignalInfo={'AMK_ActualVelocity','16','16','LE','signed','Standard','0','1','0','0','65535';'AMK_MagnetizingCurrent','48','16','LE','signed','Standard','0','1','0','0','65535';'AMK_TorqueCurrent','32','16','LE','signed','Standard','0','1','0','0','65535';'AMK_bDcOn1','12','1','LE','unsigned','Standard','0','1','0','0','1';'AMK_bDerating1','15','1','LE','unsigned','Standard','0','1','0','0','1';'AMK_bError1','9','1','LE','unsigned','Standard','0','1','0','0','1';'AMK_bInverterOn1','14','1','LE','unsigned','Standard','0','1','0','0','1';'AMK_bQuitDcOn1','11','1','LE','unsigned','Standard','0','1','0','0','1';'AMK_bQuitInverterOn1','13','1','LE','unsigned','Standard','0','1','0','0','1';'AMK_bReserve1','0','8','LE','unsigned','Standard','0','1','0','0','255';'AMK_bSystemReady1','8','1','LE','unsigned','Standard','0','1','0','0','1';'AMK_bWarn1','10','1','LE','unsigned','Standard','0','1','0','0','1'}
      settings: SourceProductBaseCode=ME,XP,VN  DataFormat=CANdb specified signals
  CAN Unpack : canmsglib/CAN Unpack  CANdbFile=D:\desktop\刘科良\HRT23赛季刘科良\CANdbc\enable.dbc  MsgList=(none)  MsgName=AMK_ActualValue1  MsgIDType=Standard (11-bit identifier)  MsgIdentifier=643  MsgLength=8  SignalInfo={'AMK_ActualVelocity','16','16','LE','signed','Standard','0','1','0','0','65535';'AMK_MagnetizingCurrent','48','16','LE','signed','Standard','0','1','0','0','65535';'AMK_TorqueCurrent','32','16','LE','signed','Standard','0','1','0','0','65535';'AMK_bDcOn1','12','1','LE','unsigned','Standard','0','1','0','0','1';'AMK_bDerating1','15','1','LE','unsigned','Standard','0','1','0','0','1';'AMK_bError1','9','1','LE','unsigned','Standard','0','1','0','0','1';'AMK_bInverterOn1','14','1','LE','unsigned','Standard','0','1','0','0','1';'AMK_bQuitDcOn1','11','1','LE','unsigned','Standard','0','1','0','0','1';'AMK_bQuitInverterOn1','13','1','LE','unsigned','Standard','0','1','0','0','1';'AMK_bReserve1','0','8','LE','unsigned','Standard','0','1','0','0','255';'AMK_bSystemReady1','8','1','LE','unsigned','Standard','0','1','0','0','1';'AMK_bWarn1','10','1','LE','unsigned','Standard','0','1','0','0','1'}  IDPort=off  TimestampPort=off  ErrorPort=off  RemotePort=off  LengthPort=off  StatusPort=off  ApplyMinMax=off
      settings: SourceProductBaseCode=ME,XP,VN  DataFormat=CANdb specified signals
  CANPackMessage : ec5744lib/RapidECU_U4B/04CANCommunication/CANPackMessage  Commented=on  datalength=8  sampletime=-1
      settings: SourceProductName=ECUCoder for MPC5744
  CANUnPackMessage : ec5744lib/RapidECU_U4B/04CANCommunication/CANUnPackMessage  datalength=8  canmessagetype=Standard(11-bit ID)  sampletime=-1
      settings: SourceProductName=ECUCoder for MPC5744
  Data Store Write : DataStoreWrite  DataStoreName=dianji_velcoity_zuoqian
  Data Store Write1 : DataStoreWrite  DataStoreName=dianji_velcoity_zuoqian1
  MATLAB Function : MATLAB Function  TreatAsAtomicUnit=on
  wires:
  msg/1 -> CANUnPackMessage/2
  CANUnPackMessage/1 -> CAN Unpack/1
  ID/1 -> CANUnPackMessage/1
  CANPackMessage/1 -> ?
  CAN Pack/1 -> CANPackMessage/1
  CAN Unpack/1 -> Data Store Write1/1, MATLAB Function/1(u)
  MATLAB Function/1(y) -> Data Store Write/1

== system ultra/RX/284 286右前/Subsystem1/Subsystem ==
  ID : Inport
  msg : Inport  Port=2
  Enable : EnablePort
  CAN Pack : canmsglib/CAN Pack  Commented=on  CANdbFile=D:\desktop\enable.dbc  MsgList=(none)  MsgName=AMK_ActualValue1  MsgIDType=Standard (11-bit identifier)  MsgIdentifier=643  MsgLength=8  Remote=off  ApplyMinMax=off  BusOutput=off  SignalInfo={'AMK_ActualVelocity','16','16','LE','signed','Standard','0','1','0','0','65535';'AMK_MagnetizingCurrent','48','16','LE','signed','Standard','0','1','0','0','65535';'AMK_TorqueCurrent','32','16','LE','signed','Standard','0','1','0','0','65535';'AMK_bDcOn1','12','1','LE','unsigned','Standard','0','1','0','0','1';'AMK_bDerating1','15','1','LE','unsigned','Standard','0','1','0','0','1';'AMK_bError1','9','1','LE','unsigned','Standard','0','1','0','0','1';'AMK_bInverterOn1','14','1','LE','unsigned','Standard','0','1','0','0','1';'AMK_bQuitDcOn1','11','1','LE','unsigned','Standard','0','1','0','0','1';'AMK_bQuitInverterOn1','13','1','LE','unsigned','Standard','0','1','0','0','1';'AMK_bReserve1','0','8','LE','unsigned','Standard','0','1','0','0','255';'AMK_bSystemReady1','8','1','LE','unsigned','Standard','0','1','0','0','1';'AMK_bWarn1','10','1','LE','unsigned','Standard','0','1','0','0','1'}
      settings: SourceProductBaseCode=ME,XP,VN  DataFormat=CANdb specified signals
  CAN Unpack : canmsglib/CAN Unpack  CANdbFile=D:\desktop\刘科良\HRT23赛季刘科良\CANdbc\enable - youqian.dbc  MsgList=(none)  MsgName=AMK_ActualValue2  MsgIDType=Standard (11-bit identifier)  MsgIdentifier=646  MsgLength=8  SignalInfo={'AMK_ErrorInfo','32','16','LE','unsigned','Standard','0','1','0','0','65535';'AMK_TempIGBT','48','16','LE','signed','Standard','0','1','0','0','65535';'AMK_TempInverter','16','16','LE','signed','Standard','0','1','0','-32768','32767';'AMK_TempMotor','0','16','LE','signed','Standard','0','1','0','0','65535'}  IDPort=off  TimestampPort=off  ErrorPort=off  RemotePort=off  LengthPort=off  StatusPort=off  ApplyMinMax=off
      settings: SourceProductBaseCode=ME,XP,VN  DataFormat=CANdb specified signals
  CANPackMessage : ec5744lib/RapidECU_U4B/04CANCommunication/CANPackMessage  Commented=on  datalength=8  sampletime=-1
      settings: SourceProductName=ECUCoder for MPC5744
  CANUnPackMessage : ec5744lib/RapidECU_U4B/04CANCommunication/CANUnPackMessage  datalength=8  canmessagetype=Standard(11-bit ID)  sampletime=-1
      settings: SourceProductName=ECUCoder for MPC5744
  wires:
  msg/1 -> CANUnPackMessage/2
  CANUnPackMessage/1 -> CAN Unpack/1
  ID/1 -> CANUnPackMessage/1
  CANPackMessage/1 -> ?
  CAN Pack/1 -> CANPackMessage/1
